simulink library "Kuka_Visual"  (R2026a)
settings: Solver=VariableStepAuto
libraries: sim3dlib x16
settings Model: Creator=shueb  LastModifiedBy=shueb

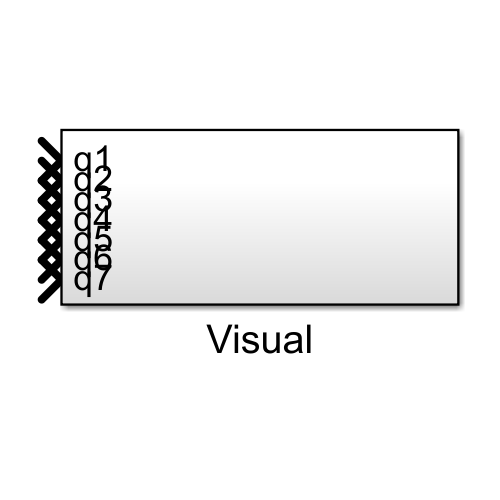
[thumbnail: Simulink's stored preview of the top-level diagram]
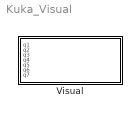
== system Kuka_Visual ==
  Visual : Subsystem

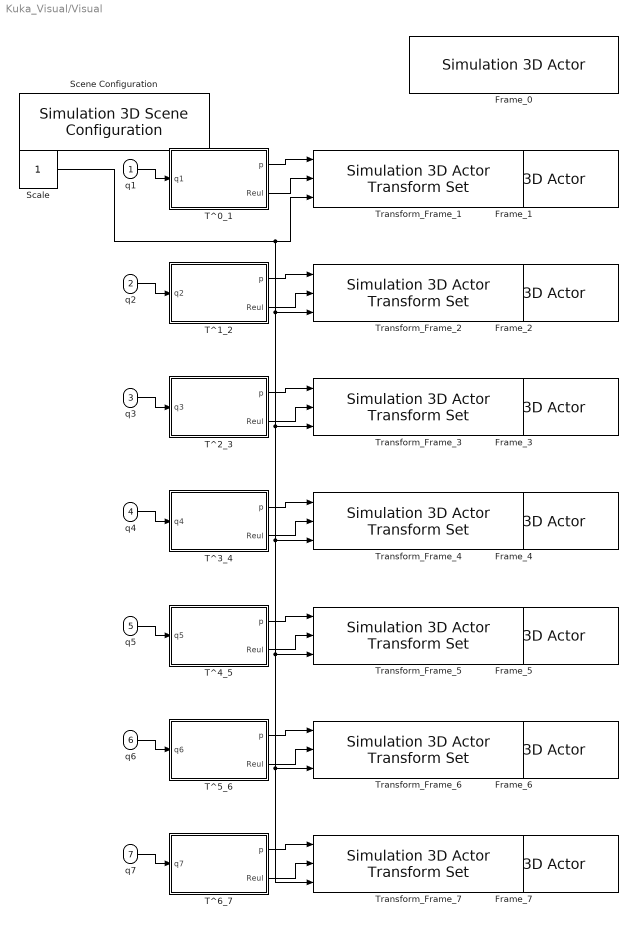
== system Kuka_Visual/Visual ==
  q1 : Inport
  q2 : Inport  Port=2
  q3 : Inport  Port=3
  q4 : Inport  Port=4
  q5 : Inport  Port=5
  q6 : Inport  Port=6
  q7 : Inport  Port=7
  Frame_0 : sim3dlib/Simulation 3D Actor  Priority=1  ActorName=Frame_0  ParentName=Scene Origin  Operation=Create at setup  InitScriptText="Actor.CoordinateSystem = \"MATLAB\";"  SampleTime=-1  Translation=[0 0 0]  Rotation=[0 0 0]  Scale=[1 1 1]  aMode=aMode  ActorType=Sim3dActor  ID=0
  Frame_1 : sim3dlib/Simulation 3D Actor  Priority=1  ActorName=Frame_1  ParentName=Frame_0  Operation=Create at setup  InitScriptText="Actor.CoordinateSystem = \"MATLAB\";"  SampleTime=-1  Translation=[0 0 0]  Rotation=[0 0 0]  Scale=[1 1 1]  aMode=aMode  ActorType=Sim3dActor  ID=0
  Frame_2 : sim3dlib/Simulation 3D Actor  Priority=1  ActorName=Frame_2  ParentName=Frame_1  Operation=Create at setup  InitScriptText="Actor.CoordinateSystem = \"MATLAB\";"  SampleTime=-1  Translation=[0 0 0]  Rotation=[0 0 0]  Scale=[1 1 1]  aMode=aMode  ActorType=Sim3dActor  ID=0
  Frame_3 : sim3dlib/Simulation 3D Actor  Priority=1  ActorName=Frame_3  ParentName=Frame_2  Operation=Create at setup  InitScriptText="Actor.CoordinateSystem = \"MATLAB\";"  SampleTime=-1  Translation=[0 0 0]  Rotation=[0 0 0]  Scale=[1 1 1]  aMode=aMode  ActorType=Sim3dActor  ID=0
  Frame_4 : sim3dlib/Simulation 3D Actor  Priority=1  ActorName=Frame_4  ParentName=Frame_3  Operation=Create at setup  InitScriptText="Actor.CoordinateSystem = \"MATLAB\";"  SampleTime=-1  Translation=[0 0 0]  Rotation=[0 0 0]  Scale=[1 1 1]  aMode=aMode  ActorType=Sim3dActor  ID=0
  Frame_5 : sim3dlib/Simulation 3D Actor  Priority=1  ActorName=Frame_5  ParentName=Frame_4  Operation=Create at setup  InitScriptText="Actor.CoordinateSystem = \"MATLAB\";"  SampleTime=-1  Translation=[0 0 0]  Rotation=[0 0 0]  Scale=[1 1 1]  aMode=aMode  ActorType=Sim3dActor  ID=0
  Frame_6 : sim3dlib/Simulation 3D Actor  Priority=1  ActorName=Frame_6  ParentName=Frame_5  Operation=Create at setup  InitScriptText="Actor.CoordinateSystem = \"MATLAB\";"  SampleTime=-1  Translation=[0 0 0]  Rotation=[0 0 0]  Scale=[1 1 1]  aMode=aMode  ActorType=Sim3dActor  ID=0
  Frame_7 : sim3dlib/Simulation 3D Actor  Priority=1  ActorName=Frame_7  ParentName=Frame_6  Operation=Create at setup  InitScriptText="Actor.CoordinateSystem = \"MATLAB\";"  SampleTime=-1  Translation=[0 0 0]  Rotation=[0 0 0]  Scale=[1 1 1]  aMode=aMode  ActorType=Sim3dActor  ID=0
  Scale : Constant
  Scene Configuration : sim3dlib/Simulation 3D Scene Configuration  Priority=0  ProjectFormat=Default Scenes  SceneDesc=Empty scene  ProjectName=C:\Program Files\MATLAB\R2026a\toolbox\shared\sim3d_projects\automotive_project_windows\UE\WindowsNoEditor\VehicleSimulation.exe  ScenePath=/Game/Maps/HwStrght  EnableOpenDRIVE=off  vehTagList={'Scene Origin', 'Custom'}  vehTag=Scene Origin  AttachedCameraRelativeTranslation=[0 0 0]  FreeCameraDefaultInitialTranslation=[-6, 0, 2]  AttachedCameraRelativeRotation=[0, -15, 0]  FreeCameraDefaultInitialRotation=[0, -15, 0]  ViewpointName=Custom  FreeCameraInitialTranslation=[0 0 0]  FreeCameraInitialRotation=[0 0 0]  OpVisEn=off  Ts=0.02  EnableWindow=on  EnableRemoteAccess=off  SimulationMode=CoSimulation  SimulateUsing=Interpreted execution  EnableAnimationRecording=off  OverrideDefaultRecording=off  AnimationRecordingFileName=sim3dAnimation.mat  AnimationRecordingInterval=[0 inf]  EnableWeather=off  SunAzimuth=90  SunAltitude=40.0  EnableGeospatialSun=off  Latitude=0  Longitude=0  Date=2023-01-01  Time=10:30:00  GeoTimeZone=-5.0  SunDaylightSaving=off  wind=1  clouds=10  EnableVolumetricClouds=off  CloudCoverage=0  CloudAltitude=6  fog=0  rain=0  RaindropsEffect=off  SnowDensity=0  EnableGeospatial=off  TilesetSource=Earth terrain  UseTrueOrigin=off  OriginHeight=200  OriginLatitude=40.744652  OriginLongitude=-73.988864  MapStyle=Aerial  AdditionalAssetIDs=[]  UseAdvancedSunSky=off  SolarTime=11  TimeZone=-5  Day=21  Month=9  Year=2022  UseDaylightSavingTime=on  DSTStartDay=10  DSTStartMonth=3  DSTEndDay=3  DSTEndMonth=11  DSTSwitchHour=2  sensorTag=MainCamera1  sensorId=1  sensorName=MainCamera1  mountLoc=Origin  offsetFlag=off  tmountOffset=[0, 0, 0]  rmountOffset=[0, 0, 0]  HorizontalResolution=1280  VerticalResolution=720  HorizontalFOV=60  mountPoint=[0 0 0]  mountOrientation=[0 0 0]  aMode=aMode  ID=1  GeoTrigger=Inactive  ViewNameList={'Custom'}  ViewTranslationList={'[0 0 0]'}  ViewRotationList={'[0 0 0]'}
  T^0_1 : MATLAB Function  TreatAsAtomicUnit=on
  T^1_2 : MATLAB Function  TreatAsAtomicUnit=on
  T^2_3 : MATLAB Function  TreatAsAtomicUnit=on
  T^3_4 : MATLAB Function  TreatAsAtomicUnit=on
  T^4_5 : MATLAB Function  TreatAsAtomicUnit=on
  T^5_6 : MATLAB Function  TreatAsAtomicUnit=on
  T^6_7 : MATLAB Function  TreatAsAtomicUnit=on
  Transform_Frame_1 : sim3dlib/Simulation 3D Actor Transform Set  Priority=-1  ActorTag=Frame_1  NumberOfParts=1  CustNumOfParts=3  CoordinateSystem=MATLAB  Translation=[0 0 0]  Rotation=[0 0 0]  Scale=[1 1 1]  Ts=-1  aMode=aMode
  Transform_Frame_2 : sim3dlib/Simulation 3D Actor Transform Set  Priority=-1  ActorTag=Frame_2  NumberOfParts=1  CustNumOfParts=3  CoordinateSystem=MATLAB  Translation=[0 0 0]  Rotation=[0 0 0]  Scale=[1 1 1]  Ts=-1  aMode=aMode
  Transform_Frame_3 : sim3dlib/Simulation 3D Actor Transform Set  Priority=-1  ActorTag=Frame_3  NumberOfParts=1  CustNumOfParts=3  CoordinateSystem=MATLAB  Translation=[0 0 0]  Rotation=[0 0 0]  Scale=[1 1 1]  Ts=-1  aMode=aMode
  Transform_Frame_4 : sim3dlib/Simulation 3D Actor Transform Set  Priority=-1  ActorTag=Frame_4  NumberOfParts=1  CustNumOfParts=3  CoordinateSystem=MATLAB  Translation=[0 0 0]  Rotation=[0 0 0]  Scale=[1 1 1]  Ts=-1  aMode=aMode
  Transform_Frame_5 : sim3dlib/Simulation 3D Actor Transform Set  Priority=-1  ActorTag=Frame_5  NumberOfParts=1  CustNumOfParts=3  CoordinateSystem=MATLAB  Translation=[0 0 0]  Rotation=[0 0 0]  Scale=[1 1 1]  Ts=-1  aMode=aMode
  Transform_Frame_6 : sim3dlib/Simulation 3D Actor Transform Set  Priority=-1  ActorTag=Frame_6  NumberOfParts=1  CustNumOfParts=3  CoordinateSystem=MATLAB  Translation=[0 0 0]  Rotation=[0 0 0]  Scale=[1 1 1]  Ts=-1  aMode=aMode
  Transform_Frame_7 : sim3dlib/Simulation 3D Actor Transform Set  Priority=-1  ActorTag=Frame_7  NumberOfParts=1  CustNumOfParts=3  CoordinateSystem=MATLAB  Translation=[0 0 0]  Rotation=[0 0 0]  Scale=[1 1 1]  Ts=-1  aMode=aMode
  wires:
  T^0_1/1(p) -> Transform_Frame_1/1
  T^0_1/2(Reul) -> Transform_Frame_1/2
  Scale/1 -> Transform_Frame_7/3, Transform_Frame_6/3, Transform_Frame_5/3, Transform_Frame_4/3, Transform_Frame_3/3, Transform_Frame_2/3, Transform_Frame_1/3
  q1/1 -> T^0_1/1(q1)
  T^1_2/1(p) -> Transform_Frame_2/1
  T^1_2/2(Reul) -> Transform_Frame_2/2
  q2/1 -> T^1_2/1(q2)
  T^2_3/1(p) -> Transform_Frame_3/1
  T^2_3/2(Reul) -> Transform_Frame_3/2
  q3/1 -> T^2_3/1(q3)
  T^3_4/1(p) -> Transform_Frame_4/1
  T^3_4/2(Reul) -> Transform_Frame_4/2
  q4/1 -> T^3_4/1(q4)
  T^4_5/1(p) -> Transform_Frame_5/1
  T^4_5/2(Reul) -> Transform_Frame_5/2
  q5/1 -> T^4_5/1(q5)
  T^5_6/1(p) -> Transform_Frame_6/1
  T^5_6/2(Reul) -> Transform_Frame_6/2
  q6/1 -> T^5_6/1(q6)
  T^6_7/1(p) -> Transform_Frame_7/1
  T^6_7/2(Reul) -> Transform_Frame_7/2
  q7/1 -> T^6_7/1(q7)

== matlab function Kuka_Visual/Visual/T^0_1 ==
  data: q1 input; p output; Reul output
function [p,Reul] = T_0_1(q1)
%#codegen

%    This function was generated by the Symbolic Math Toolbox version 26.1.
%    15-May-2026 08:52:26

% q1 = complex(q1);  % if required to enforce complex operations
p = [0.0,0.0,0.0];
if nargout > 1
    Reul = [pi./2.0,0.0,q1];
end
end

== matlab function Kuka_Visual/Visual/T^2_3 ==
  data: q3 input; p output; Reul output
function [p,Reul] = T_2_3(q3)
%#codegen

%    This function was generated by the Symbolic Math Toolbox version 26.1.
%    15-May-2026 08:52:27

% q3 = complex(q3);  % if required to enforce complex operations
p = [0.0,0.0,2.0./5.0];
if nargout > 1
    Reul = [pi.*(-1.0./2.0),0.0,q3];
end
end

== matlab function Kuka_Visual/Visual/T^3_4 ==
  data: q4 input; p output; Reul output
function [p,Reul] = T_3_4(q4)
%#codegen

%    This function was generated by the Symbolic Math Toolbox version 26.1.
%    15-May-2026 08:52:28

% q4 = complex(q4);  % if required to enforce complex operations
p = [0.0,0.0,0.0];
if nargout > 1
    Reul = [pi./2.0,0.0,q4];
end
end

== matlab function Kuka_Visual/Visual/T^4_5 ==
  data: q5 input; p output; Reul output
function [p,Reul] = T_4_5(q5)
%#codegen

%    This function was generated by the Symbolic Math Toolbox version 26.1.
%    15-May-2026 08:52:28

% q5 = complex(q5);  % if required to enforce complex operations
p = [0.0,0.0,2.0./5.0];
if nargout > 1
    Reul = [pi./2.0,0.0,q5];
end
end

== matlab function Kuka_Visual/Visual/T^5_6 ==
  data: q6 input; p output; Reul output
function [p,Reul] = T_5_6(q6)
%#codegen

%    This function was generated by the Symbolic Math Toolbox version 26.1.
%    15-May-2026 08:52:29

% q6 = complex(q6);  % if required to enforce complex operations
p = [0.0,0.0,0.0];
if nargout > 1
    Reul = [pi.*(-1.0./2.0),0.0,q6];
end
end

== matlab function Kuka_Visual/Visual/T^6_7 ==
  data: q7 input; p output; Reul output
function [p,Reul] = T_6_7(q7)
%#codegen

%    This function was generated by the Symbolic Math Toolbox version 26.1.
%    15-May-2026 08:52:30

% q7 = complex(q7);  % if required to enforce complex operations
p = [0.0,0.0,6.3e+1./5.0e+2];
if nargout > 1
    Reul = [0.0,0.0,q7];
end
end

== matlab function Kuka_Visual/Visual/T^1_2 ==
  data: q2 input; p output; Reul output
function [p,Reul] = T_1_2(q2)
%#codegen

%    This function was generated by the Symbolic Math Toolbox version 26.1.
%    15-May-2026 08:52:26

% q2 = complex(q2);  % if required to enforce complex operations
p = [0.0,0.0,0.0];
if nargout > 1
    Reul = [pi.*(-1.0./2.0),0.0,q2];
end
end
